simulink model "LorentsAttractor"  (R2019b)
settings: Solver=VariableStepAuto  StartTime=0.0  StopTime=100  MaxStep=0.01  RelTol=1e-3
PreLoadFcn:
  | rho = 24
  | x0 = [1 1 1]
  | x1 = [1.01 1 1]
  | x2 = [1 1.01 1]
StopFcn:
  | plot3(out.X(:,1),out.X(:,2),out.X(:,3),'b-')
  | hold on
  | plot3(out.X1(:,1),out.X1(:,2),out.X1(:,3),'r-')
  | plot3(out.X2(:,1),out.X2(:,2),out.X2(:,3),'g-')
  | hold off
  | grid
PauseFcn:
  | plot3(out.X(:,1),out.X(:,2),out.X(:,3))
  | grid
settings Model: Creator=francescopolcri  LastModifiedBy=francescopolcri

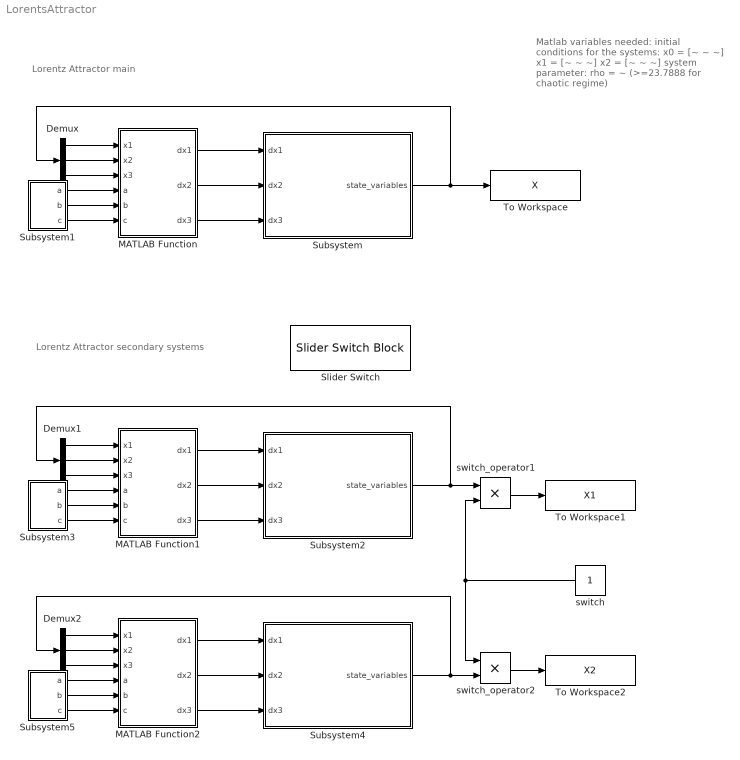
== system LorentsAttractor ==
  note: Matlab variables needed:
      | initial conditions for the systems:
      | x0 = [~ ~ ~]
      | x1 = [~ ~ ~]
      | x2 = [~ ~ ~]
      | system parameter:
      | rho = ~ (>=23.7888 for chaotic regime)
  note: Lorentz Attractor main
  note: Lorentz Attractor secondary systems
  Demux : Demux  Outputs=3
  Demux1 : Demux  Outputs=3
  Demux2 : Demux  Outputs=3
  MATLAB Function : MATLAB Function  TreatAsAtomicUnit=on
  MATLAB Function1 : MATLAB Function  TreatAsAtomicUnit=on
  MATLAB Function2 : MATLAB Function  TreatAsAtomicUnit=on
  Slider Switch : SliderSwitchBlock
      settings: Values={{'Off', 'On'}, [0 1]}
  Subsystem : Subsystem
  Subsystem1 : Subsystem
  Subsystem2 : Subsystem
  Subsystem3 : Subsystem
  Subsystem4 : Subsystem
  Subsystem5 : Subsystem
  To Workspace : ToWorkspace  VariableName=X  SampleTime=-1
  To Workspace1 : ToWorkspace  VariableName=X1  SampleTime=-1
  To Workspace2 : ToWorkspace  VariableName=X2  SampleTime=-1
  "switch " : Constant
  switch_operator1 : Product
  switch_operator2 : Product
  wires:
  MATLAB Function/3(dx3) -> Subsystem/3(dx3)
  MATLAB Function/2(dx2) -> Subsystem/2(dx2)
  MATLAB Function/1(dx1) -> Subsystem/1(dx1)
  Subsystem/1(state_variables) -> Demux/1, To Workspace/1
  Demux/1 -> MATLAB Function/1(x1)
  Demux/2 -> MATLAB Function/2(x2)
  Demux/3 -> MATLAB Function/3(x3)
  Subsystem1/1(a) -> MATLAB Function/4(a)
  Subsystem1/2(b) -> MATLAB Function/5(b)
  Subsystem1/3(c) -> MATLAB Function/6(c)
  Subsystem2/1(state_variables) -> switch_operator1/1, Demux1/1
  MATLAB Function1/1(dx1) -> Subsystem2/1(dx1)
  Subsystem3/2(b) -> MATLAB Function1/5(b)
  Subsystem3/3(c) -> MATLAB Function1/6(c)
  Demux1/1 -> MATLAB Function1/1(x1)
  MATLAB Function1/2(dx2) -> Subsystem2/2(dx2)
  Demux1/2 -> MATLAB Function1/2(x2)
  MATLAB Function1/3(dx3) -> Subsystem2/3(dx3)
  Demux1/3 -> MATLAB Function1/3(x3)
  Subsystem3/1(a) -> MATLAB Function1/4(a)
  MATLAB Function2/1(dx1) -> Subsystem4/1(dx1)
  Subsystem5/3(c) -> MATLAB Function2/6(c)
  Subsystem5/2(b) -> MATLAB Function2/5(b)
  Subsystem5/1(a) -> MATLAB Function2/4(a)
  Demux2/2 -> MATLAB Function2/2(x2)
  Demux2/3 -> MATLAB Function2/3(x3)
  MATLAB Function2/2(dx2) -> Subsystem4/2(dx2)
  MATLAB Function2/3(dx3) -> Subsystem4/3(dx3)
  Demux2/1 -> MATLAB Function2/1(x1)
  Subsystem4/1(state_variables) -> switch_operator2/2, Demux2/1
  switch_operator2/1 -> To Workspace2/1
  switch_operator1/1 -> To Workspace1/1
  "switch "/1 -> switch_operator2/1, switch_operator1/2

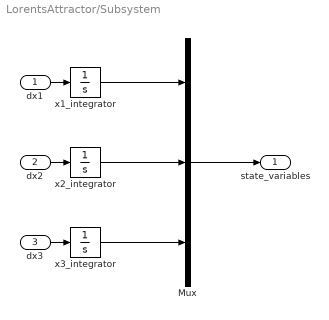
== system LorentsAttractor/Subsystem ==
  dx1 : Inport
  dx2 : Inport  Port=2
  dx3 : Inport  Port=3
  Mux : Mux  Inputs=3
  x1_integrator : Integrator  InitialCondition=x0(1)
  x2_integrator : Integrator  InitialCondition=x0(2)
  "x3_integrator " : Integrator  InitialCondition=x0(3)
  state_variables : Outport
  wires:
  dx1/1 -> x1_integrator/1
  dx2/1 -> x2_integrator/1
  dx3/1 -> "x3_integrator "/1
  x1_integrator/1 -> Mux/1
  "x3_integrator "/1 -> Mux/3
  x2_integrator/1 -> Mux/2
  Mux/1 -> state_variables/1

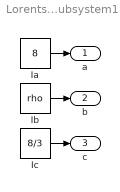
== system LorentsAttractor/Subsystem1 ==
  Ia : Constant  Value=8
  Ib : Constant  Value=rho
  Ic : Constant  Value=8/3
  a : Outport
  b : Outport  Port=2
  c : Outport  Port=3
  wires:
  Ic/1 -> c/1
  Ia/1 -> a/1
  Ib/1 -> b/1

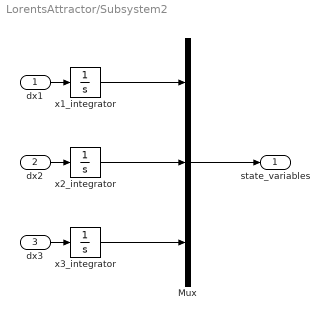
== system LorentsAttractor/Subsystem2 ==
  dx1 : Inport
  dx2 : Inport  Port=2
  dx3 : Inport  Port=3
  Mux : Mux  Inputs=3
  x1_integrator : Integrator  InitialCondition=x1(1)
  x2_integrator : Integrator  InitialCondition=x1(2)
  "x3_integrator " : Integrator  InitialCondition=x1(3)
  state_variables : Outport
  wires:
  dx1/1 -> x1_integrator/1
  dx2/1 -> x2_integrator/1
  dx3/1 -> "x3_integrator "/1
  x1_integrator/1 -> Mux/1
  "x3_integrator "/1 -> Mux/3
  x2_integrator/1 -> Mux/2
  Mux/1 -> state_variables/1

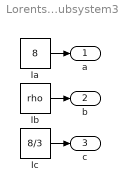
== system LorentsAttractor/Subsystem3 ==
  Ia : Constant  Value=8
  Ib : Constant  Value=rho
  Ic : Constant  Value=8/3
  a : Outport
  b : Outport  Port=2
  c : Outport  Port=3
  wires:
  Ic/1 -> c/1
  Ia/1 -> a/1
  Ib/1 -> b/1

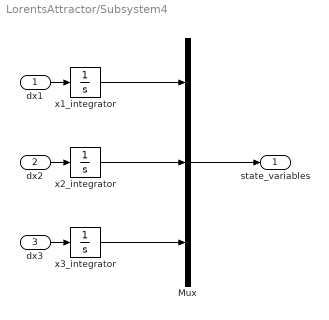
== system LorentsAttractor/Subsystem4 ==
  dx1 : Inport
  dx2 : Inport  Port=2
  dx3 : Inport  Port=3
  Mux : Mux  Inputs=3
  x1_integrator : Integrator  InitialCondition=x2(1)
  x2_integrator : Integrator  InitialCondition=x2(2)
  "x3_integrator " : Integrator  InitialCondition=x2(3)
  state_variables : Outport
  wires:
  dx1/1 -> x1_integrator/1
  dx2/1 -> x2_integrator/1
  dx3/1 -> "x3_integrator "/1
  x1_integrator/1 -> Mux/1
  "x3_integrator "/1 -> Mux/3
  x2_integrator/1 -> Mux/2
  Mux/1 -> state_variables/1

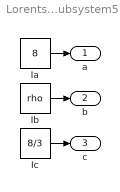
== system LorentsAttractor/Subsystem5 ==
  Ia : Constant  Value=8
  Ib : Constant  Value=rho
  Ic : Constant  Value=8/3
  a : Outport
  b : Outport  Port=2
  c : Outport  Port=3
  wires:
  Ic/1 -> c/1
  Ia/1 -> a/1
  Ib/1 -> b/1

== matlab function LorentsAttractor/MATLAB Function1 ==
  data: x1 input; dx1 output; x2 input; x3 input; a input; b input; dx2 output; dx3 output; c input
function [dx1,dx2,dx3] = fcn(x1,x2,x3,a,b,c)
dx1 = a*(x2-x1);
dx2 = b*x1-x1*x3-x2;
dx3 = x1*x2-c*x3;

== matlab function LorentsAttractor/MATLAB Function ==
  data: x1 input; dx1 output; x2 input; x3 input; a input; b input; dx2 output; dx3 output; c input
function [dx1,dx2,dx3] = fcn(x1,x2,x3,a,b,c)
dx1 = a*(x2-x1);
dx2 = b*x1-x1*x3-x2;
dx3 = x1*x2-c*x3;

== matlab function LorentsAttractor/MATLAB Function2 ==
  data: x1 input; dx1 output; x2 input; x3 input; a input; b input; dx2 output; dx3 output; c input
function [dx1,dx2,dx3] = fcn(x1,x2,x3,a,b,c)
dx1 = a*(x2-x1);
dx2 = b*x1-x1*x3-x2;
dx3 = x1*x2-c*x3;
